simulink model "sf_cycle_error_fix"  (R2017b)
settings: Solver=ode45  StartTime=0.0  StopTime=10.0  RelTol=1e-3  EnableMultiTasking=on
settings Model: FPTRunName=Active  ExtModeTrigMode=oneshot  ExtModeArmWhenConnect=off  ExtModeAutoUpdateStatusClock=off  Creator=The MathWorks, Inc.  LastModifiedBy=The MathWorks, Inc.
settings DataIOCC: SaveFormat=Array
settings OptimizationCC: BooleanDataType=off  ExpressionDepthLimit=2147483647  InitFltsAndDblsToZero=on  LifeSpan=inf
settings DebuggingCC: SaveWithParameterizedLinksMsg=none  UnderspecifiedInitializationDetection=Classic  MergeDetectMultiDrivingBlocksExec=none  SignalResolutionControl=TryResolveAllWithWarning  MultiTaskDSMMsg=warning  MultiTaskCondExecSysMsg=none  FcnCallInpInsideContextMsg=warning  StateNameClashWarn=warning  StrictBusMsg=None  SFUnexpectedBacktrackingDiag=warning  SFNoUnconditionalDefaultTransitionDiag=warning  SFExecutionAtInitializationDiag=none
settings HardwareCC: ProdBitPerPointer=32  ProdBitPerSizeT=32  ProdBitPerPtrDiffT=32  ProdLargestAtomicFloat=None  ProdIntDivRoundTo=Undefined  ProdEndianess=Unspecified  ProdWordSize=32  ProdHWDeviceType=32-bit Generic  TargetUnknown=on
settings ModelReferenceCC: PropagateSignalLabelsOutOfModel=off
settings SFSimCC: SimParseCustomCode=off
settings CodeAppCC: StateflowObjectComments=on
settings GRTTargetCC: TargetFcnLib=ansi_tfl_tmw.mat  TargetLangStandard=C89/C90 (ANSI)  GeneratePreprocessorConditionals=Disable all  CombineOutputUpdateFcns=off  GRTInterface=on
settings ConfigComp: CovMetricSettings=dcmtr  CovHtmlReporting=on  CovSaveCumulativeToWorkspaceVar=on  CovSaveSingleToWorkspaceVar=on  CovExternalEMLEnable=off  CovSFcnEnable=off

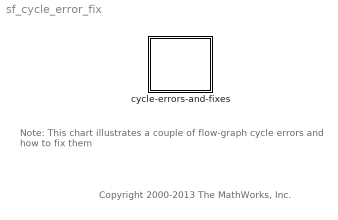
== system sf_cycle_error_fix ==
  note: Note: This chart illustrates a couple of flow-graph
      | cycle errors and  how to fix them
  note: Copyright 2000-2013 The MathWorks, Inc.
  cycle-errors-and-fixes : Stateflow chart  TreatAsAtomicUnit=on

== stateflow chart sf_cycle_error_fix/cycle-errors-and-fixes ==
  state Note: [group]
    The following diagrams illustrate a couple of flow-graph cycle errors and  how to fix them
  state Fix1: [group]
    We incorporate the negation of condition c1
    into the transition containing c2 such that the
    resulting diagram is functionally equivalent
    and has an unconditional path out of the loop
    to termination.
    (default) -> (junction 26)
    (junction 27) -> (junction 26) [order 1] : [!c1 && c2]
    (junction 26) -> (junction 27) : {action2;}
    (junction 27) -> (junction 28) [order 2]
  state Error1: [group]
    The bottom junction in the loop
    does not have an unconditional
    path to termination
    (default) -> (junction 23)
    (junction 24) -> (junction 23) [order 2] : [c2]
    (junction 23) -> (junction 24) : {action1;}
    (junction 24) -> (junction 25) [order 1] : [c1]
  state Error2: [group]
    The top junction in the loop
    does not have an unconditional
    path to termination
    (default) -> (junction 29)
    (junction 30) -> (junction 29) [order 1] : [c2]
    (junction 29) -> (junction 30) : [c1]{action1;}
    (junction 30) -> (junction 31) [order 2] : {action2;}
  state Fix2: [group]
    We create an unconditional transition from
    the top junction to the terminal junction.
    Once again, this is functionally equivalent
    (default) -> (junction 32)
    (junction 33) -> (junction 32) [order 1] : [c2]
    (junction 32) -> (junction 34) [order 2]
    (junction 32) -> (junction 33) [order 1] : [c1]{action1;}
    (junction 33) -> (junction 34) [order 2] : {action2;}
